simulink model "PIDGainSchedCSTRExampleModel"  (R2015b)
settings: Solver=ode23t  StartTime=0.0  StopTime=200  RelTol=1e-3
PreLoadFcn:
  | load PIDGainSchedExample.mat
model workspace (MAT data in the model file):
  op_snapshot1 : opcond.OperatingPoint (value not decoded)
values from neighbouring files (symbols this model uses):
  C = [2 3 4 5 6 7 8 9]    [linearizePID.m]
undefined symbols (not defined in the file or in its folder): Controllers, D, I, N, P, sigbuilder_block
libraries: simulink x1
settings Model: Creator=The MathWorks, Inc.  LastModifiedBy=gnardelli
settings DataIOCC: ExternalInput=getinputstruct(op_snapshot1)  InitialState=getstatestruct(op_snapshot1)  LoadExternalInput=on  LoadInitialState=on  SaveFormat=Array
settings OptimizationCC: ExpressionDepthLimit=2147483647
settings DebuggingCC: AlgebraicLoopMsg=none  UnderspecifiedInitializationDetection=Classic  MergeDetectMultiDrivingBlocksExec=none  FcnCallInpInsideContextMsg=UseLocalSettings  UnconnectedInputMsg=none  UnconnectedOutputMsg=none  UnconnectedLineMsg=none  StateNameClashWarn=warning
settings HardwareCC: ProdBitPerPointer=32  ProdLargestAtomicFloat=None  ProdIntDivRoundTo=Undefined  ProdEndianess=Unspecified  ProdWordSize=32  ProdHWDeviceType=32-bit Generic
settings GRTTargetCC: GeneratePreprocessorConditionals=Disable all  CombineOutputUpdateFcns=off  GRTInterface=on
settings ConfigComp: CovModelRefEnable=Off

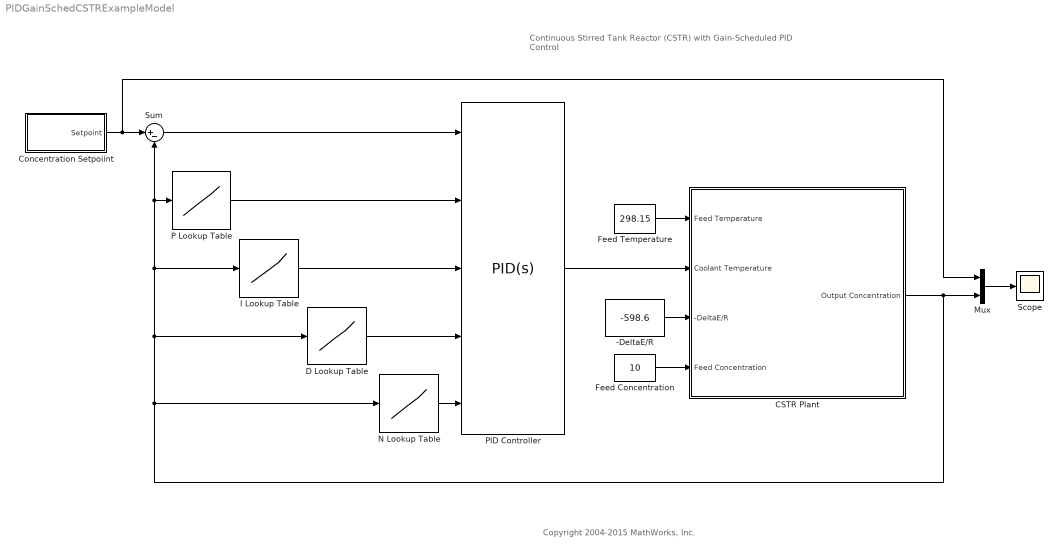
== system PIDGainSchedCSTRExampleModel ==
  note: Copyright 2004-2015 MathWorks, Inc.
  note: Continuous Stirred Tank Reactor (CSTR)
      | with Gain-Scheduled PID Control
  -DeltaE/R : Constant  Value=-598.6  SampleTime=0
  CSTR Plant : Subsystem
  Concentration Setpoiint : Subsystem  Tag=STV Subsys  LoadFcn=sigbuilder_block('load');  StartFcn=sigbuilder_block('start');  StopFcn=sigbuilder_block('stop');  ClipboardFcn=sigbuilder_block('clipboard');  mask(Sigbuilder block){}
      mask help: Simulink:masks:SigbuilderBlock_MD
      mask init:
      | if ~strcmp(get_param(bdroot(gcbh),'SimulationStatus'),'stopped') tuvar = sigbuilder_block('maskInit'); end
      settings: CopyFcn=sigbuilder_block('copy');  DeleteFcn=sigbuilder_block('delete');  ModelCloseFcn=sigbuilder_block('modelClose');  PreSaveFcn=sigbuilder_block('preSave');  PauseFcn=sigbuilder_block('pause');  ContinueFcn=sigbuilder_block('continue');  NameChangeFcn=sigbuilder_block('namechange');  OpenFcn=sigbuilder_block('open',[437.6 199.2 550.4 400 ]);  CloseFcn=sigbuilder_block('close');
      mask Display: plot(0, 0, 100, 100,[2, 2, 32, 32, 2], [68, 8, 8, 68, 68],[32, 2], [38, 38], [32, 19, 2],[53, 60, 44], [32, 17, 17, 2],[16, 16, 31, 31]);txt = getActiveGroup(gcbh);text(2, 100, txt,'verticalAlignment', 'top');
  D Lookup Table : Lookup_n-D  NumberOfTableDimensions=1  BreakpointsForDimension1=C  Table=Controllers.Kd  ExtrapMethod=Clip  UseLastTableValue=on  InternalRulePriority=Speed  RndMeth=Simplest  InputSameDT=on
  Feed Concentration : Constant  Value=10  SampleTime=0
  Feed Temperature : Constant  Value=298.15  SampleTime=0
  I Lookup Table : Lookup_n-D  NumberOfTableDimensions=1  BreakpointsForDimension1=C  Table=[-401.9513925319188,-171.36070627079224,-138.89414480407828,-151.12830857659688,-203.85341578161567,-315.57142478751496,-612.8686897168064,-1604.08119678907]  ExtrapMethod=Clip  UseLastTableValue=on  InternalRulePriority=Speed  RndMeth=Simplest  InputSameDT=on
  Mux : Mux  Inputs=2
  N Lookup Table : Lookup_n-D  NumberOfTableDimensions=1  BreakpointsForDimension1=C  Table=1./(Controllers.Tf)  ExtrapMethod=Clip  UseLastTableValue=on  InternalRulePriority=Speed  RndMeth=Simplest  InputSameDT=on
  P Lookup Table : Lookup_n-D  NumberOfTableDimensions=1  BreakpointsForDimension1=C  Table=Controllers.Kp  ExtrapMethod=Clip  UseLastTableValue=on  InternalRulePriority=Speed  RndMeth=Simplest  InputSameDT=on
  PID Controller : simulink/Continuous/PID Controller  Controller=PID  TimeDomain=Continuous-time  SampleTime=-1  IntegratorMethod=Forward Euler  FilterMethod=Forward Euler  Form=Parallel  UseFilter=on  ControllerParametersSource=external  P=P(1)  I=I(1)  D=D(1)  N=N(1)  InitialConditionSource=internal  InitialConditionForIntegrator=0  InitialConditionForFilter=0  ExternalReset=none  LimitOutput=off  UpperSaturationLimit=350  LowerSaturationLimit=250  LinearizeAsGain=on  AntiWindupMode=none  Kb=1  TrackingMode=off  Kt=1  PParamMin=[]  PParamMax=[]  IParamMin=[]  IParamMax=[]  DParamMin=[]  DParamMax=[]  NParamMin=[]  NParamMax=[]  KbParamMin=[]  KbParamMax=[]  KtParamMin=[]  KtParamMax=[]  POutMin=[]  POutMax=[]  IOutMin=[]  IOutMax=[]  DOutMin=[]  DOutMax=[]  NOutMin=[]  NOutMax=[]  KbOutMin=[]  KbOutMax=[]  KtOutMin=[]  KtOutMax=[]  IntegratorOutMin=[]  IntegratorOutMax=[]  FilterOutMin=[]  FilterOutMax=[]  SumOutMin=[]  SumOutMax=[]  SumI1OutMin=[]  SumI1OutMax=[]  SumI2OutMin=[]  SumI2OutMax=[]  SumI3OutMin=[]  SumI3OutMax=[]  SumDOutMin=[]  SumDOutMax=[]  SaturationOutMin=[]  SaturationOutMax=[]  IntegratorContinuousStateAttributes=''  IntegratorStateMustResolveToSignalObject=off  IntegratorRTWStateStorageClass=Auto  FilterContinuousStateAttributes=''  FilterStateMustResolveToSignalObject=off  FilterRTWStateStorageClass=Auto  DifferentiatorICPrevScaledInput=0  DifferentiatorOutMin=[]  DifferentiatorOutMax=[]
  Scope : Scope
  Sum : Sum  Inputs=|+-
  wires:
  Feed Temperature/1 -> CSTR Plant/1(Feed Temperature)
  -DeltaE/R/1 -> CSTR Plant/3(-DeltaE/R)
  Feed Concentration/1 -> CSTR Plant/4(Feed Concentration)
  CSTR Plant/1(Output Concentration) -> Mux/2, Sum/2, P Lookup Table/1, I Lookup Table/1, D Lookup Table/1, N Lookup Table/1
  PID Controller/1 -> CSTR Plant/2(Coolant Temperature)
  Sum/1 -> PID Controller/1
  P Lookup Table/1 -> PID Controller/2
  I Lookup Table/1 -> PID Controller/3
  D Lookup Table/1 -> PID Controller/4
  N Lookup Table/1 -> PID Controller/5
  Concentration Setpoiint/1(Setpoint) -> Mux/1, Sum/1
  Mux/1 -> Scope/1

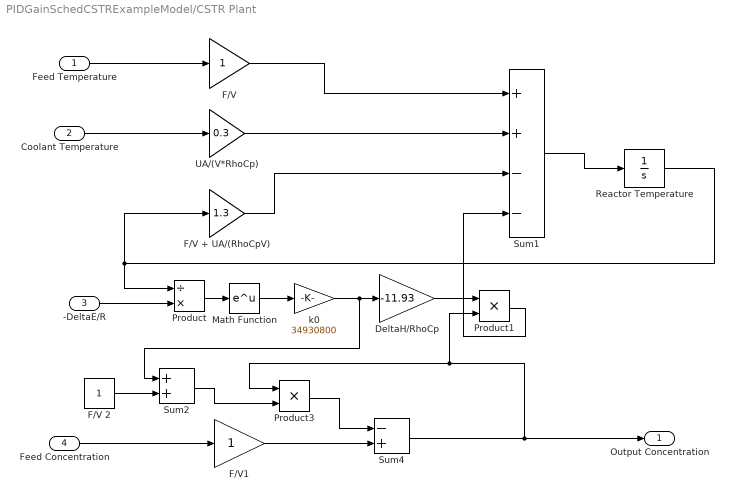
== system PIDGainSchedCSTRExampleModel/CSTR Plant ==
  Feed Temperature : Inport
  Coolant Temperature : Inport  Port=2
  -DeltaE/R : Inport  Port=3
  Feed Concentration : Inport  Port=4
  DeltaH/RhoCp : Gain  Gain=-11.93  SaturateOnIntegerOverflow=on  OutDataTypeStr=Inherit: Same as input  ParamDataTypeStr=Inherit: Same as input
  F/V : Gain  SaturateOnIntegerOverflow=on  OutDataTypeStr=Inherit: Same as input  ParamDataTypeStr=Inherit: Same as input
  F/V + UA/(RhoCpV) : Gain  Gain=1.3  SaturateOnIntegerOverflow=on  OutDataTypeStr=Inherit: Same as input  ParamDataTypeStr=Inherit: Same as input
  F/V 2 : Constant  SampleTime=0
  F/V1 : Gain  SaturateOnIntegerOverflow=on  OutDataTypeStr=Inherit: Same as input  ParamDataTypeStr=Inherit: Same as input
  Math Function : Math  SaturateOnIntegerOverflow=on
  Product : Product  Inputs=/*  SaturateOnIntegerOverflow=on  RndMeth=Zero  InputSameDT=on  OutDataTypeStr=Inherit: Same as first input
  Product1 : Product  SaturateOnIntegerOverflow=on  RndMeth=Zero  InputSameDT=on  OutDataTypeStr=Inherit: Same as first input
  Product3 : Product  SaturateOnIntegerOverflow=on  RndMeth=Zero  InputSameDT=on  OutDataTypeStr=Inherit: Same as first input
  Reactor Temperature : Integrator  InitialCondition=300  LimitOutput=on  LowerSaturationLimit=0
  Sum1 : Sum  Inputs=++--  SaturateOnIntegerOverflow=on  InputSameDT=on  OutDataTypeStr=Inherit: Same as first input
  Sum2 : Sum  SaturateOnIntegerOverflow=on  InputSameDT=on  OutDataTypeStr=Inherit: Same as first input
  Sum4 : Sum  Inputs=-+  SaturateOnIntegerOverflow=on  InputSameDT=on  OutDataTypeStr=Inherit: Same as first input
  UA/(V*RhoCp) : Gain  Gain=0.3  SaturateOnIntegerOverflow=on  OutDataTypeStr=Inherit: Same as input  ParamDataTypeStr=Inherit: Same as input
  k0 : Gain  Gain=34930800  SaturateOnIntegerOverflow=on  OutDataTypeStr=Inherit: Same as input  ParamDataTypeStr=Inherit: Same as input
  Output Concentration : Outport
  wires:
  Sum2/1 -> Product3/2
  Coolant Temperature/1 -> UA/(V*RhoCp)/1
  Feed Concentration/1 -> F/V1/1
  Feed Temperature/1 -> F/V/1
  F/V1/1 -> Sum4/2
  F/V 2/1 -> Sum2/2
  Sum4/1 -> Output Concentration/1, Product1/2, Product3/1
  Product3/1 -> Sum4/1
  -DeltaE/R/1 -> Product/2
  k0/1 -> Sum2/1, DeltaH/RhoCp/1
  Product1/1 -> Sum1/4
  DeltaH/RhoCp/1 -> Product1/1
  Math Function/1 -> k0/1
  Product/1 -> Math Function/1
  F/V + UA/(RhoCpV)/1 -> Sum1/3
  UA/(V*RhoCp)/1 -> Sum1/2
  Reactor Temperature/1 -> F/V + UA/(RhoCpV)/1, Product/1
  Sum1/1 -> Reactor Temperature/1
  F/V/1 -> Sum1/1

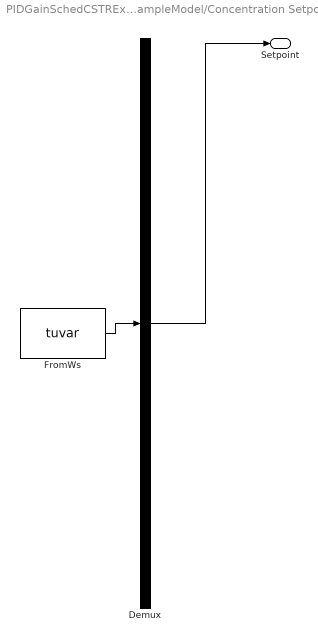
== system PIDGainSchedCSTRExampleModel/Concentration Setpoiint ==
  Demux : Demux  Tag=STV Demux  Outputs=1
  FromWs : FromWorkspace  Tag=STV FromWs  VariableName=tuvar  SampleTime=0
      SigBuilderData=|
      | common.afterFinalStr = 'Extrapolate'
      | common.sampleTime = 0
      | dataSet.timeRange = [0 200]
      | dataSet.name = 'Group 1'
      | sbobj.Groups.Name = 'Group 1'
      | sbobj.Groups.Signals.Name = 'Setpoint'
      | sbobj.Groups.Signals.XData = [0 10 10 20 20 30 30 40 40 50 50 60 60 70 70 80 80 90 90 100 100 110 110 120 120 130 130 140 140 160 160.5 180 180.5 200]
      | sbobj.Groups.Signals.YData = [9 9 7.98 7.98 7 7 6 6 5.02 5.02 4.02 4.02 3 3 2 2 3 3 4 4 5 5 6 6 7 7 8 8 9 9 2 2 9 9]
      | sbobj.Groups.TimeRange = [0 200]
  Setpoint : Outport  Tag=STV Outport
  wires:
  Demux/1 -> Setpoint/1
  FromWs/1 -> Demux/1
